simulink library "Brake_Control_ABS"  (R2025a)
settings: Solver=VariableStepAuto  StartTime=0.0  StopTime=10.0  RelTol=1e-3
undefined symbols (not defined in the file): abs_tire_radiusF, abs_tire_radiusR
libraries: Brake_Control_ABS_Valve x4
Description:
  | Simscape Vehicle Templates Library
  | 
  | Copyright 2018-2025 The MathWorks, Inc.
settings Model: Creator=smiller  LastModifiedBy=smiller
settings OptimizationCC: ReuseModelBlockBuffer=off
settings ModelReferenceCC: EnableRefExpFcnMdlSchedulingChecks=on
settings RTWCC: GPUComputeCapability=3.5

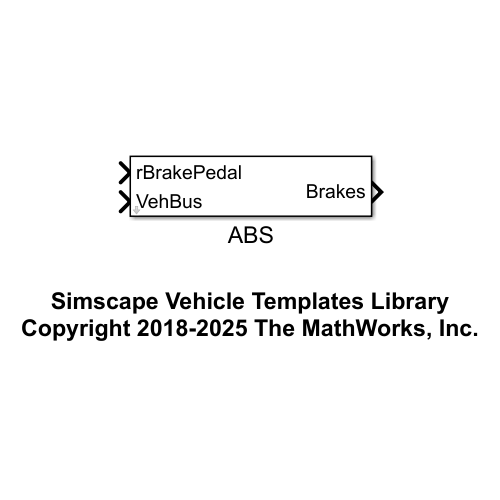
[thumbnail: Simulink's stored preview of the top-level diagram]
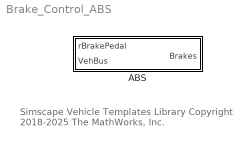
== system Brake_Control_ABS ==
  note: Simscape Vehicle Templates Library
      | Copyright 2018-2025 The MathWorks, Inc.
  ABS : Subsystem  VariantControl=ABS  mask{abs_tire_radiusF=abs_tire_radiusF, abs_tire_radiusR=abs_tire_radiusR}
      mask prompts: abs_tire_radiusF "Tire Radius Front (m)"; abs_tire_radiusR "Tire Radius Rear (m)"

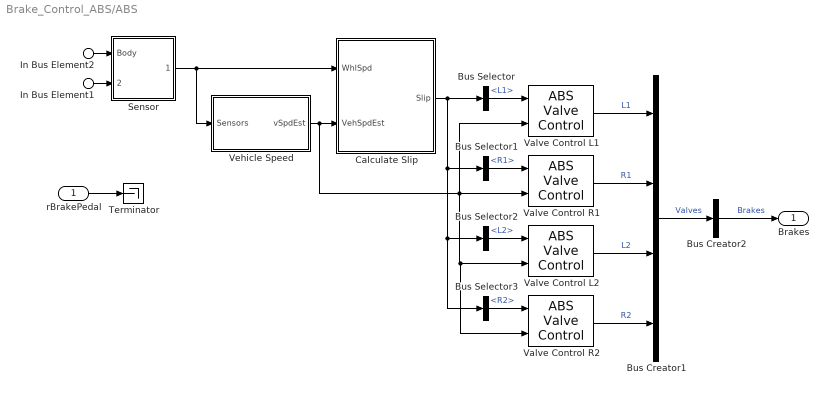
== system Brake_Control_ABS/ABS ==
  rBrakePedal : Inport
  In Bus Element1 : Inport  Port=2  PortName=VehBus  Element=Chassis
  In Bus Element2 : Inport  Port=2  PortName=VehBus  Element=Chassis.Body.CG
  Bus Creator1 : BusCreator  Inputs=4
  Bus Creator2 : BusCreator  Inputs=1
  Bus Selector : BusSelector  OutputSignals=L1
  Bus Selector1 : BusSelector  OutputSignals=R1
  Bus Selector2 : BusSelector  OutputSignals=L2
  Bus Selector3 : BusSelector  OutputSignals=R2
  Calculate Slip : Subsystem
  Sensor : Subsystem
  Terminator : Terminator
  Valve Control L1 : Brake_Control_ABS_Valve/ABS Valve Control  SystemSampleTime=-1  VariantActivationTime=update diagram  EmptyChoice=off  PassThrough=off  PassThroughVariantControl=(default)  EmptyChoiceVariantControl=(default)  AllowFlexibleInterface=on  Latency=0  AutoFrameSizeCalculation=off
  Valve Control L2 : Brake_Control_ABS_Valve/ABS Valve Control  SystemSampleTime=-1  VariantActivationTime=update diagram  EmptyChoice=off  PassThrough=off  PassThroughVariantControl=(default)  EmptyChoiceVariantControl=(default)  AllowFlexibleInterface=on  Latency=0  AutoFrameSizeCalculation=off
  Valve Control R1 : Brake_Control_ABS_Valve/ABS Valve Control  SystemSampleTime=-1  VariantActivationTime=update diagram  EmptyChoice=off  PassThrough=off  PassThroughVariantControl=(default)  EmptyChoiceVariantControl=(default)  AllowFlexibleInterface=on  Latency=0  AutoFrameSizeCalculation=off
  Valve Control R2 : Brake_Control_ABS_Valve/ABS Valve Control  SystemSampleTime=-1  VariantActivationTime=update diagram  EmptyChoice=off  PassThrough=off  PassThroughVariantControl=(default)  EmptyChoiceVariantControl=(default)  AllowFlexibleInterface=on  Latency=0  AutoFrameSizeCalculation=off
  Vehicle Speed : Subsystem
  Brakes : Outport  VectorParamsAs1DForOutWhenUnconnected=off
  wires:
  In Bus Element2/1 -> Sensor/1(Body)
  In Bus Element1/1 -> Sensor/2(WhlSpd)
  Bus Creator2/1 -> Brakes/1  "Brakes"
  Bus Selector1/1 -> Valve Control R1/1  "<R1>"
  Valve Control L1/1 -> Bus Creator1/1  "L1"
  Calculate Slip/1(Slip) -> Bus Selector/1, Bus Selector1/1, Bus Selector2/1, Bus Selector3/1
  Bus Selector/1 -> Valve Control L1/1  "<L1>"
  Bus Selector3/1 -> Valve Control R2/1  "<R2>"
  Valve Control L2/1 -> Bus Creator1/3  "L2"
  Valve Control R2/1 -> Bus Creator1/4  "R2"
  Valve Control R1/1 -> Bus Creator1/2  "R1"
  Bus Selector2/1 -> Valve Control L2/1  "<L2>"
  Bus Creator1/1 -> Bus Creator2/1  "Valves"
  Sensor/1(GroundSpd) -> Calculate Slip/1(WhlSpd), Vehicle Speed/1(Sensors)
  Vehicle Speed/1(vSpdEst) -> Calculate Slip/2(VehSpdEst), Valve Control L1/2, Valve Control R1/2, Valve Control L2/2, Valve Control R2/2
  rBrakePedal/1 -> Terminator/1

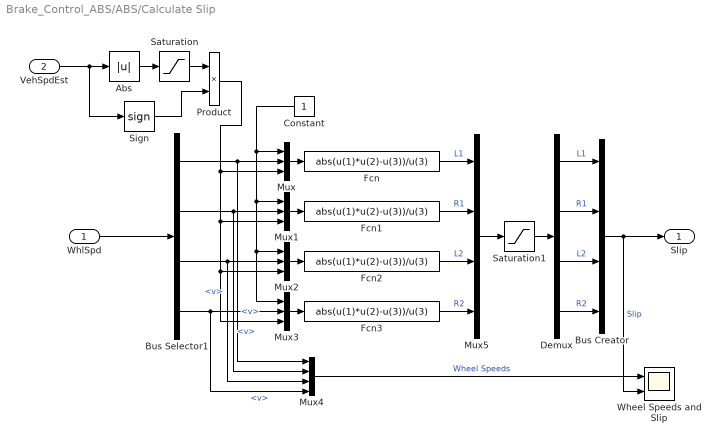
== system Brake_Control_ABS/ABS/Calculate Slip ==
  WhlSpd : Inport
  VehSpdEst : Inport  Port=2
  Abs : Abs  ZeroCross=off  SaturateOnIntegerOverflow=off
  Bus Creator : BusCreator  Inputs=4
  Bus Selector1 : BusSelector  OutputSignals=L1.v,R1.v,L2.v,R2.v
  Constant : Constant
  Demux : Demux
  Fcn{,1..3} (4 alike) : Fcn  Expr=abs(u(1)*u(2)-u(3))/u(3)
  Mux{,1..3} (4 alike) : Mux  Inputs=3
  Mux4 : Mux
  Mux5 : Mux
  Product : Product
  Saturation : Saturate  UpperLimit=inf  LowerLimit=eps  ZeroCross=off
  Saturation1 : Saturate  UpperLimit=1  LowerLimit=0
  Sign : Signum  ZeroCross=off
  Wheel Speeds and Slip : Scope  NumInputPorts=2
      settings: ActiveDisplayYMinimum=-11.64241  ActiveDisplayYMaximum=114.01232  DataLoggingVariableName=ScopeData2
  Slip : Outport  VectorParamsAs1DForOutWhenUnconnected=off
  wires:
  Fcn3/1 -> Mux5/4  "R2"
  Fcn2/1 -> Mux5/3  "L2"
  Fcn1/1 -> Mux5/2  "R1"
  Fcn/1 -> Mux5/1  "L1"
  Saturation1/1 -> Demux/1
  Mux5/1 -> Saturation1/1
  Mux4/1 -> Wheel Speeds and Slip/1  "Wheel Speeds"
  Mux3/1 -> Fcn3/1
  Mux2/1 -> Fcn2/1
  Mux1/1 -> Fcn1/1
  Mux/1 -> Fcn/1
  Sign/1 -> Product/2
  Saturation/1 -> Product/1
  Abs/1 -> Saturation/1
  Product/1 -> Mux/3, Mux1/3, Mux2/3, Mux3/3
  Bus Creator/1 -> Slip/1, Wheel Speeds and Slip/2  "Slip"
  Demux/4 -> Bus Creator/4  "R2"
  Demux/3 -> Bus Creator/3  "L2"
  Demux/2 -> Bus Creator/2  "R1"
  Demux/1 -> Bus Creator/1  "L1"
  VehSpdEst/1 -> Abs/1, Sign/1
  Constant/1 -> Mux2/1, Mux3/1, Mux1/1, Mux/1
  Bus Selector1/3 -> Mux2/2, Mux4/3  "<v>"
  Bus Selector1/1 -> Mux/2, Mux4/1  "<v>"
  Bus Selector1/4 -> Mux3/2, Mux4/4  "<v>"
  Bus Selector1/2 -> Mux1/2, Mux4/2  "<v>"
  WhlSpd/1 -> Bus Selector1/1

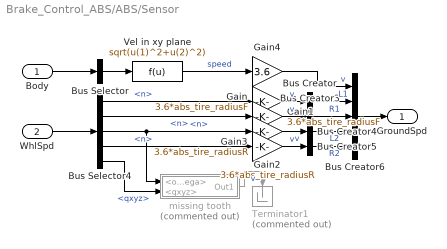
== system Brake_Control_ABS/ABS/Sensor ==
  Body : Inport
  WhlSpd : Inport  Port=2
  Bus Creator{,3..5} (4 alike) : BusCreator  Inputs=1
  Bus Creator6 : BusCreator  Inputs=5
  Bus Selector : BusSelector  OutputSignals=vx,vy  OutputAsBus=on
  Bus Selector4 : BusSelector  OutputSignals=WhlL1.n,WhlR1.n,WhlL2.n,WhlR2.n,WhlL2.qxyz
  Gain : Gain  Gain=3.6*abs_tire_radiusF
  Gain1 : Gain  Gain=3.6*abs_tire_radiusF
  Gain2 : Gain  Gain=3.6*abs_tire_radiusR
  Gain3 : Gain  Gain=3.6*abs_tire_radiusR
  Gain4 : Gain  Gain=3.6
  Terminator1 : Terminator  Commented=on
  Vel in xy plane : Fcn  Expr=sqrt(u(1)^2+u(2)^2)
  missing tooth : Subsystem  Commented=on
  GroundSpd : Outport  VectorParamsAs1DForOutWhenUnconnected=off
  wires:
  Bus Selector/1 -> Vel in xy plane/1
  Vel in xy plane/1 -> Gain4/1  "speed"
  Bus Creator6/1 -> GroundSpd/1
  WhlSpd/1 -> Bus Selector4/1
  Bus Selector4/4 -> Gain3/1  "<n>"
  Bus Selector4/1 -> Gain/1  "<n>"
  Gain4/1 -> Bus Creator6/1  "v"
  Bus Creator3/1 -> Bus Creator6/3  "R1"
  Body/1 -> Bus Selector/1
  Gain/1 -> Bus Creator/1  "v"
  Bus Selector4/3 -> missing tooth/1(<omega>), Gain2/1  "<n>"
  Bus Creator4/1 -> Bus Creator6/4  "L2"
  Bus Selector4/2 -> Gain1/1  "<n>"
  Bus Creator/1 -> Bus Creator6/2  "L1"
  Gain3/1 -> Bus Creator5/1  "v"
  Bus Creator5/1 -> Bus Creator6/5  "R2"
  Bus Selector4/5 -> missing tooth/2(<qxyz>)  "<qxyz>"
  Gain2/1 -> Bus Creator4/1  "v"
  missing tooth/1(Out1) -> Terminator1/1  "v"
  Gain1/1 -> Bus Creator3/1  "v"

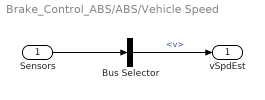
== system Brake_Control_ABS/ABS/Vehicle Speed ==
  Sensors : Inport
  Bus Selector : BusSelector  OutputSignals=v
  vSpdEst : Outport  VectorParamsAs1DForOutWhenUnconnected=off
  wires:
  Bus Selector/1 -> vSpdEst/1  "<v>"
  Sensors/1 -> Bus Selector/1

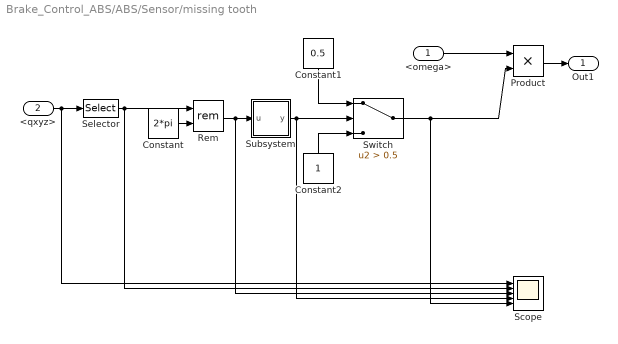
== system Brake_Control_ABS/ABS/Sensor/missing tooth ==
  <omega> : Inport
  <qxyz> : Inport  Port=2
  Constant : Constant  Value=2*pi
  Constant1 : Constant  Value=0.5
  Constant2 : Constant
  Product : Product
  Rem : Math  Operator=rem  SignedPower=on
  Scope : Scope  NumInputPorts=5
      settings: ActiveDisplayYMinimum=-41.32335  ActiveDisplayYMaximum=259.55855  DataLoggingVariableName=ScopeData2
  Selector : Selector  InputPortWidth=3  IndexOptions=Index vector (dialog)  Indices=[2]  OutputSizes=1
  Subsystem : Subsystem  mask{int_limit_upper=25/48*2*pi, int_limit_lower=22/48*2*pi}
      mask prompts: int_limit_upper "Upper Limit"; int_limit_lower "Lower Limit"
      mask TypeOptions int_limit_upper: Upper Limit/Value
      mask TypeOptions int_limit_lower: Lower Limit/Value
  Switch : Switch  Criteria=u2 > Threshold  Threshold=0.5  SaturateOnIntegerOverflow=off  InputSameDT=off
  Out1 : Outport  VectorParamsAs1DForOutWhenUnconnected=off
  wires:
  Product/1 -> Out1/1
  <omega>/1 -> Product/1
  Constant2/1 -> Switch/3
  Constant1/1 -> Switch/1
  Switch/1 -> Product/2, Scope/5
  Subsystem/1(y) -> Switch/2, Scope/4
  Selector/1 -> Rem/1, Scope/2
  Rem/1 -> Subsystem/1(u), Scope/3
  Constant/1 -> Rem/2
  <qxyz>/1 -> Selector/1, Scope/1

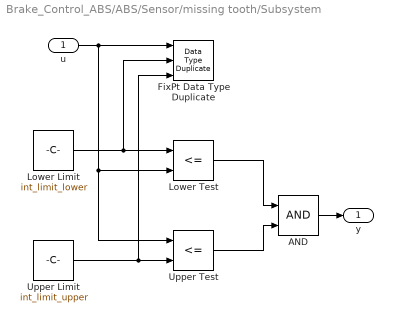
== system Brake_Control_ABS/ABS/Sensor/missing tooth/Subsystem ==
  u : Inport
  AND : Logic  AllPortsSameDT=off  OutDataTypeStr=boolean
  FixPt Data Type Duplicate : DataTypeDuplicate  DisableCoverage=on  NumInputPorts=3
  Lower Limit : Constant  DisableCoverage=on  Value=int_limit_lower  OutDataTypeStr=Inherit: Inherit via back propagation
  Lower Test : RelationalOperator  DisableCoverage=on  Operator=<=  OutDataTypeStr=boolean  InputSameDT=off
  Upper Limit : Constant  DisableCoverage=on  Value=int_limit_upper  OutDataTypeStr=Inherit: Inherit via back propagation
  Upper Test : RelationalOperator  DisableCoverage=on  Operator=<=  OutDataTypeStr=boolean  InputSameDT=off
  y : Outport  VectorParamsAs1DForOutWhenUnconnected=off
  wires:
  Lower Test/1 -> AND/1
  Upper Test/1 -> AND/2
  AND/1 -> y/1
  u/1 -> FixPt Data Type Duplicate/1, Lower Test/2, Upper Test/1
  Upper Limit/1 -> Upper Test/2, FixPt Data Type Duplicate/3
  Lower Limit/1 -> Lower Test/1, FixPt Data Type Duplicate/2
